simulink model "main"  (R2017b)
settings: Solver=FixedStepAuto  StartTime=0.0  StopTime=250  FixedStep=Ts  RelTol=1e-3
values from neighbouring files (symbols this model uses):
  dz = -0.1690    (= -0.169)    [prepareWorkspace.m]
  K = antisway.lqr()    [prepareWorkspace.m]
  omega_l = 4*2*pi    (= 25.1327412287)    [prepareWorkspace.m]
  omega_q = 1*2*pi    (= 6.28318530718)    [prepareWorkspace.m]
  Ts = 0.005    [prepareWorkspace.m]
  zeta_l = 0.7    [prepareWorkspace.m]
  zeta_q = 0.7    [prepareWorkspace.m]
undefined symbols (not defined in the file or in its folder): DiscIntNeverNeededParam, lambda, P0, Q, R, sigma, w0, x0
libraries: hydro x2
settings Model: Creator=motionlab  LastModifiedBy=motionlab
settings OptimizationCC: LocalBlockOutputs=off
settings DebuggingCC: BusObjectLabelMismatch=error
settings RTWCC: SystemTargetFile=TwinCAT.tlc  GenCodeOnly=on  MakeCommand=make_tct  TemplateMakefile=tct_msbuild.tmf  Description=TwinCAT Target  GenerateReport=on  TargetLang=C++
settings STFCustomTargetCC: TargetLangStandard=C++03 (ISO)  CompOptLevelCompliant=on  MATLABClassNameForMDSCustomization=Simulink.SoftwareTarget.TargetSpecificTriggerConfigurationBase  SystemTargetFile=TwinCAT.tlc
settings ConfigComp: PLC_TargetIDE=twincat3  PLC_GenerateReusableCode=on  PLC_InlineNamedConstant=on  PLC_ReuseMLFcnVariable=on  PLC_GenerateReport=off  PLC_LaunchReport=off

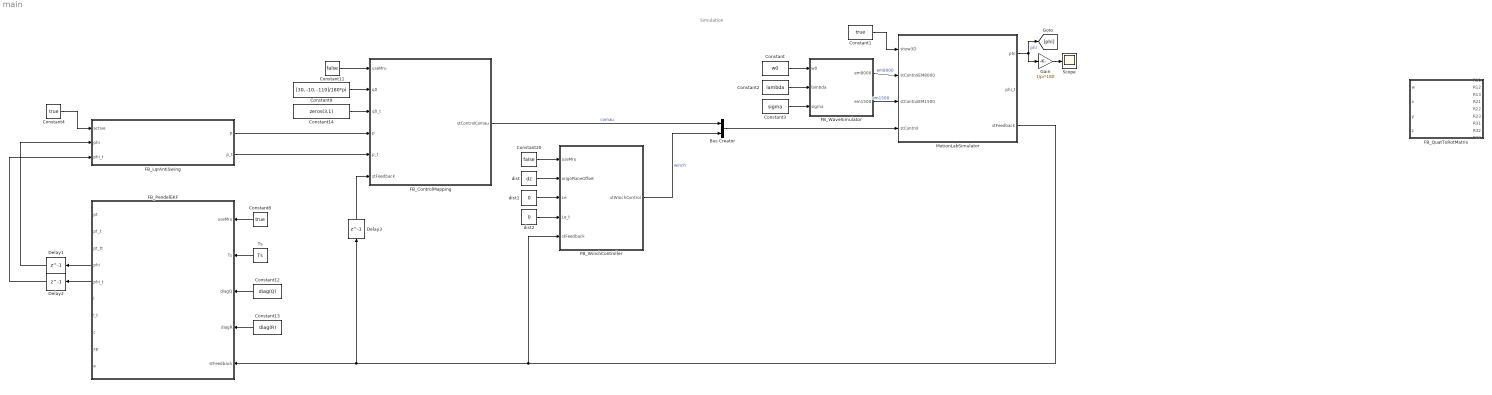
== system main ==
  note: Simulation
  Bus Creator : BusCreator  Inputs=2  OutDataTypeStr=Bus: ST_Control
  Constant : Constant  Value=w0
  Constant1 : Constant  Value=true
  Constant11 : Constant  Value=false
  Constant12 : Constant  Value=diag(Q)
  Constant13 : Constant  Value=diag(R)
  Constant14 : Constant  Value=zeros(3,1)
  Constant2 : Constant  Value=lambda
  Constant20 : Constant  Value=false
  Constant3 : Constant  Value=sigma
  Constant4 : Constant  Value=true
  Constant8 : Constant  Value=true
  Constant9 : Constant  Value=[30, -10, -110]/180*pi
  Delay1 : Delay  DelayLength=1
  Delay2 : Delay  DelayLength=1
  Delay3 : Delay  DelayLength=1
  FB_ControlMapping : MATLAB Function  TreatAsAtomicUnit=on
  FB_LqrAntiSwing : Subsystem  mask{lqrK=K, lqrMax=0.4}
      mask prompts: lqrK "LQR Gain"; lqrMax "LQR Saturation"
  FB_PendelEKF : Subsystem  TreatAsAtomicUnit=on  mask{ekfX0=x0}
      mask prompts: ekfX0 "x0"
      mask DialogControl Container3 Prompt: EKF Parmeters
  FB_QuatToRotMatrix : MATLAB Function  TreatAsAtomicUnit=on
  FB_WaveSimulator : Subsystem  TreatAsAtomicUnit=on
  FB_WinchController : Subsystem  TreatAsAtomicUnit=on
  Gain : Gain  Gain=1/pi*180
  MotionLabSimulator : Subsystem  mask{w_joints=omega_q, zeta_joints=zeta_q, w_winch=omega_l, zeta_winch=zeta_l, dz=dz, c=0.5, enableMruNoise=false}
      mask prompts: w_joints "omega [rad]"; zeta_joints "zeta [-]"; w_winch "omega [rad]"; zeta_winch "zeta [-]"; enableMruNoise "Enable"
      mask DialogControl ParameterGroupVar Prompt: Robot Joint Dynamics
      mask DialogControl Container3 Prompt: Winch Dynamics
      mask DialogControl Container4 Prompt: Ship Deck Offset From {b2}
      mask DialogControl Container5 Prompt: Pendulum Paramaters
      mask DialogControl Container6 Prompt: MRU Noise Simulation
  Scope : Scope
  Ts : Constant  Value=Ts
  dist : Constant  Value=dz
  dist1 : Constant  Value=0
  dist2 : Constant  Value=0
  wires:
  Constant1/1 -> MotionLabSimulator/1(show3D)
  Constant/1 -> FB_WaveSimulator/1(w0)
  Constant2/1 -> FB_WaveSimulator/2(lambda)
  Constant3/1 -> FB_WaveSimulator/3(sigma)
  MotionLabSimulator/1(phi) -> Gain/1, [phi]  "phi"
  Gain/1 -> Scope/1
  Constant20/1 -> FB_WinchController/1(useMru)
  dist/1 -> FB_WinchController/2(origoPlaneOffset)
  dist1/1 -> FB_WinchController/3(Le)
  FB_WaveSimulator/1(em8000) -> MotionLabSimulator/2(stControlEM8000)  "em8000"
  FB_WaveSimulator/2(em1500) -> MotionLabSimulator/3(stControlEM1500)  "em1500"
  Bus Creator/1 -> MotionLabSimulator/4(stControl)
  Constant9/1 -> FB_ControlMapping/2(q0)
  Constant11/1 -> FB_ControlMapping/1(useMru)
  Constant14/1 -> FB_ControlMapping/3(q0_t)
  FB_ControlMapping/1(stControlComau) -> Bus Creator/1  "comau"
  FB_WinchController/1(stWinchControl) -> Bus Creator/2  "winch"
  dist2/1 -> FB_WinchController/4(Le_t)
  MotionLabSimulator/3(stFeedback) -> FB_WinchController/5(stFeedback), Delay3/1, FB_PendelEKF/5(stFeedback)
  Delay3/1 -> FB_ControlMapping/6(stFeedback)
  FB_PendelEKF/5(phi_t) -> Delay2/1
  Constant8/1 -> FB_PendelEKF/1(useMru)
  Ts/1 -> FB_PendelEKF/2(Ts)
  FB_PendelEKF/4(phi) -> Delay1/1
  Constant12/1 -> FB_PendelEKF/3(diagQ)
  Constant13/1 -> FB_PendelEKF/4(diagR)
  Delay1/1 -> FB_LqrAntiSwing/2(phi)
  Delay2/1 -> FB_LqrAntiSwing/3(phi_t)
  Constant4/1 -> FB_LqrAntiSwing/1(active)
  FB_LqrAntiSwing/1(p) -> FB_ControlMapping/4(p)
  FB_LqrAntiSwing/2(p_t) -> FB_ControlMapping/5(p_t)

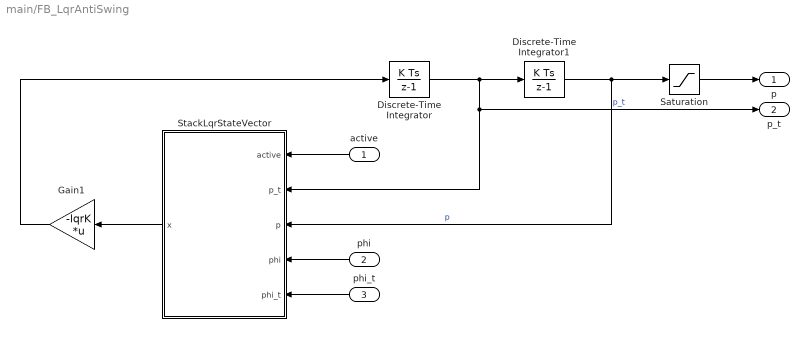
== system main/FB_LqrAntiSwing ==
  active : Inport
  phi : Inport  Port=2
  phi_t : Inport  Port=3
  Discrete-Time Integrator : DiscreteIntegrator  InitialCondition=zeros(3,1)  InitialConditionSetting=State (most efficient)  SampleTime=-1  ICPrevOutput=DiscIntNeverNeededParam  ICPrevScaledInput=DiscIntNeverNeededParam
  Discrete-Time Integrator1 : DiscreteIntegrator  InitialCondition=zeros(3,1)  InitialConditionSetting=State (most efficient)  SampleTime=-1  ICPrevOutput=DiscIntNeverNeededParam  ICPrevScaledInput=DiscIntNeverNeededParam
  Gain1 : Gain  Gain=-lqrK  Multiplication=Matrix(K*u)
  Saturation : Saturate  UpperLimit=abs(lqrMax)  LowerLimit=-abs(lqrMax)
  StackLqrStateVector : MATLAB Function  TreatAsAtomicUnit=on
  p : Outport
  p_t : Outport  Port=2
  wires:
  StackLqrStateVector/1(x) -> Gain1/1
  Gain1/1 -> Discrete-Time Integrator/1
  active/1 -> StackLqrStateVector/1(active)
  Discrete-Time Integrator1/1 -> StackLqrStateVector/3(p), Saturation/1  "p"
  Saturation/1 -> p/1
  Discrete-Time Integrator/1 -> Discrete-Time Integrator1/1, p_t/1, StackLqrStateVector/2(p_t)  "p_t"
  phi/1 -> StackLqrStateVector/4(phi)
  phi_t/1 -> StackLqrStateVector/5(phi_t)

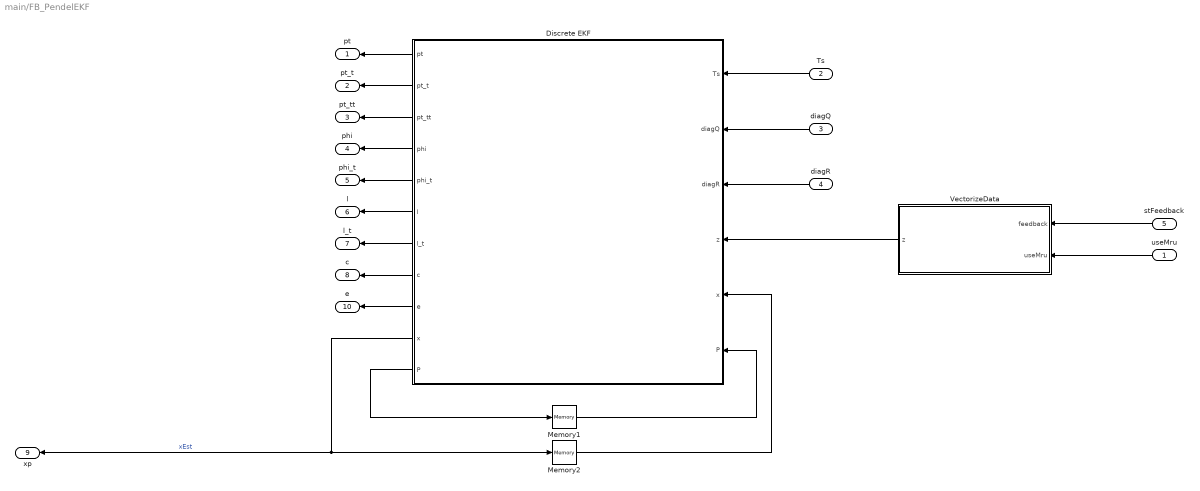
== system main/FB_PendelEKF ==
  useMru : Inport
  Ts : Inport  Port=2
  diagQ : Inport  Port=3
  diagR : Inport  Port=4
  stFeedback : Inport  Port=5  OutDataTypeStr=Bus: ST_Feedback
  Discrete EKF : MATLAB Function  TreatAsAtomicUnit=on
  Memory1 : Memory  InitialCondition=P0
  Memory2 : Memory  InitialCondition=ekfX0
  VectorizeData : MATLAB Function  TreatAsAtomicUnit=on
  pt : Outport
  pt_t : Outport  Port=2
  pt_tt : Outport  Port=3
  phi : Outport  Port=4
  phi_t : Outport  Port=5
  l : Outport  Port=6
  l_t : Outport  Port=7
  c : Outport  Port=8
  xp : Outport  Port=9
  e : Outport  Port=10
  wires:
  VectorizeData/1(z) -> Discrete EKF/4(z)
  Memory2/1 -> Discrete EKF/5("x ")
  Discrete EKF/11(P) -> Memory1/1
  Memory1/1 -> Discrete EKF/6("P ")
  diagR/1 -> Discrete EKF/3(diagR)
  diagQ/1 -> Discrete EKF/2(diagQ)
  Ts/1 -> Discrete EKF/1(Ts)
  Discrete EKF/10(x) -> xp/1, Memory2/1  "xEst"
  stFeedback/1 -> VectorizeData/1(feedback)
  useMru/1 -> VectorizeData/2(useMru)
  Discrete EKF/4(phi) -> phi/1
  Discrete EKF/5(phi_t) -> phi_t/1
  Discrete EKF/1(pt) -> pt/1
  Discrete EKF/2(pt_t) -> pt_t/1
  Discrete EKF/3(pt_tt) -> pt_tt/1
  Discrete EKF/6(l) -> l/1
  Discrete EKF/7(l_t) -> l_t/1
  Discrete EKF/8(c) -> c/1
  Discrete EKF/9(e) -> e/1

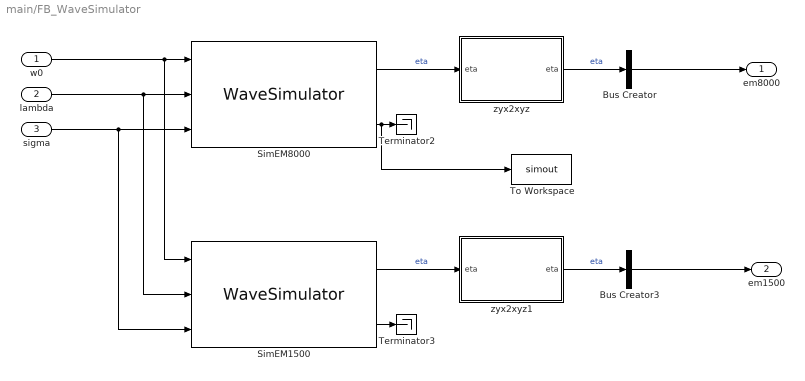
== system main/FB_WaveSimulator ==
  w0 : Inport
  lambda : Inport  Port=2
  sigma : Inport  Port=3
  Bus Creator : BusCreator  Inputs=1  OutDataTypeStr=Bus: ST_ControlStewart
  Bus Creator3 : BusCreator  Inputs=1  OutDataTypeStr=Bus: ST_ControlStewart
  SimEM1500 : hydro/WaveSimulator  poles=-30  seed=[5000,400,0,9000,150,42]  K1=1e4  K2=1e4  K3=1e8  K4=1e7  K5=1e8  K6=1e3  maxOutput=[0.1, 0.1, 0.3, 5/180*pi, 5/180*pi, 5/180*pi]  limitK=zeros(6,1)
      settings: SourceProductName=Hydro Library
  SimEM8000 : hydro/WaveSimulator  poles=-30  seed=[0,20,500,9000,400,200]  K1=1e4  K2=1e4  K3=1e8  K4=1e7  K5=1e8  K6=1e3  maxOutput=[0.1, 0.1, 0.4, 5/180*pi, 5/180*pi, 5/180*pi]  limitK=zeros(6,1)
      settings: SourceProductName=Hydro Library
  Terminator2 : Terminator
  Terminator3 : Terminator
  To Workspace : ToWorkspace  VariableName=simout  SaveFormat=Timeseries  SampleTime=-1
  zyx2xyz : MATLAB Function  TreatAsAtomicUnit=on
  zyx2xyz1 : MATLAB Function  TreatAsAtomicUnit=on
  em8000 : Outport
  em1500 : Outport  Port=2
  wires:
  zyx2xyz/1(eta) -> Bus Creator/1  "eta"
  Bus Creator3/1 -> em1500/1
  Bus Creator/1 -> em8000/1
  zyx2xyz1/1(eta) -> Bus Creator3/1  "eta"
  SimEM1500/1 -> zyx2xyz1/1("eta ")  "eta"
  SimEM8000/2 -> To Workspace/1, Terminator2/1
  SimEM8000/1 -> zyx2xyz/1("eta ")  "eta"
  SimEM1500/2 -> Terminator3/1
  w0/1 -> SimEM8000/1, SimEM1500/1
  lambda/1 -> SimEM8000/2, SimEM1500/2
  sigma/1 -> SimEM8000/3, SimEM1500/3

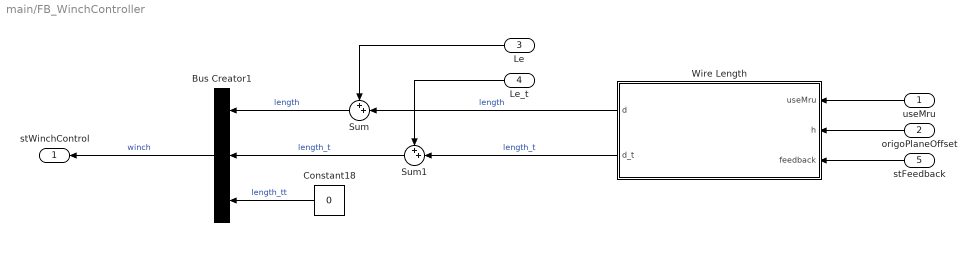
== system main/FB_WinchController ==
  useMru : Inport
  origoPlaneOffset : Inport  Port=2
  Le : Inport  Port=3
  Le_t : Inport  Port=4
  stFeedback : Inport  Port=5
  Bus Creator1 : BusCreator  Inputs=3  OutDataTypeStr=Bus: ST_ControlWinch
  Constant18 : Constant  Value=0
  Sum : Sum  Inputs=++|
  Sum1 : Sum  Inputs=++|
  Wire Length : MATLAB Function  TreatAsAtomicUnit=on
  stWinchControl : Outport
  wires:
  Bus Creator1/1 -> stWinchControl/1  "winch"
  useMru/1 -> Wire Length/1(useMru)
  origoPlaneOffset/1 -> Wire Length/2(h)
  Constant18/1 -> Bus Creator1/3  "length_tt"
  Sum/1 -> Bus Creator1/1  "length"
  Wire Length/1(d) -> Sum/2  "length"
  Le/1 -> Sum/1
  stFeedback/1 -> Wire Length/3(feedback)
  Sum1/1 -> Bus Creator1/2  "length_t"
  Wire Length/2(d_t) -> Sum1/2  "length_t"
  Le_t/1 -> Sum1/1

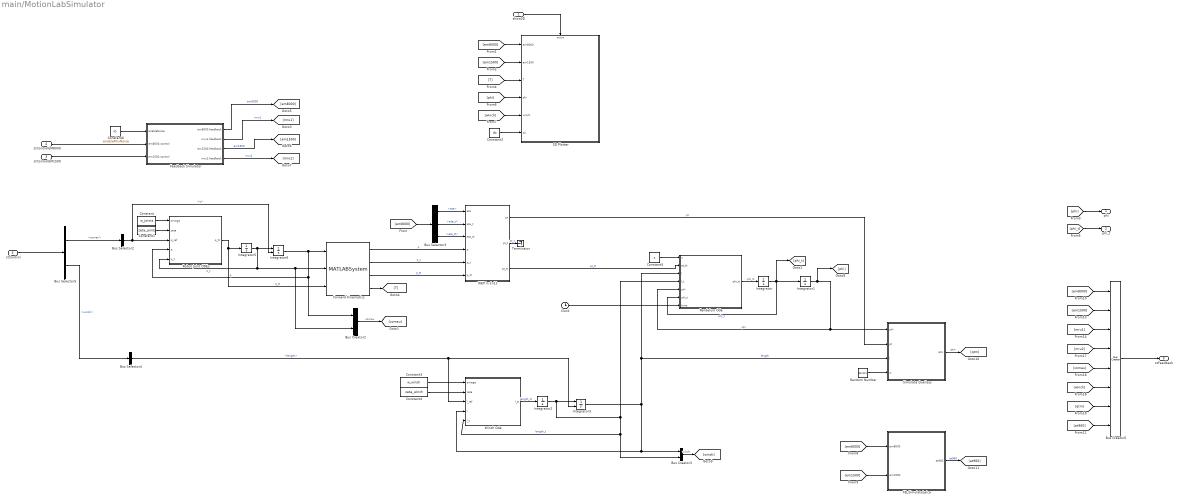
== system main/MotionLabSimulator ==
  show3D : Inport
  stControlEM8000 : Inport  Port=2  OutDataTypeStr=Bus: ST_ControlStewart
  stControlEM1500 : Inport  Port=3  OutDataTypeStr=Bus: ST_ControlStewart
  stControl : Inport  Port=4  OutDataTypeStr=Bus: ST_Control
  3D Plotter : Subsystem
  Bus Creator2 : BusCreator  Inputs=2  OutDataTypeStr=Bus: ST_FeedbackComau
  Bus Creator3 : BusCreator  Inputs=2  OutDataTypeStr=Bus: ST_FeedbackWinch
  Bus Creator5 : BusCreator  Inputs=8  OutDataTypeStr=Bus: ST_Feedback
  Bus Selector2 : BusSelector  OutputSignals=q
  Bus Selector3 : BusSelector  OutputSignals=eta,eta_t,eta_tt
  Bus Selector4 : BusSelector  OutputSignals=length
  Bus Selector5 : BusSelector  OutputSignals=comau,winch
  Clock : Clock
  Constant : Constant  Value=w_joints
  Constant1 : Constant  Value=zeta_joints
  Constant2 : Constant  Value=dz
  Constant3 : Constant  Value=w_winch
  Constant4 : Constant  Value=zeta_winch
  Constant5 : Constant  Value=c
  Constant6 : Constant  Value=enableMruNoise
  FB_SimulateLeica : MATLAB Function  TreatAsAtomicUnit=on
  Feedback Simulator : Subsystem
  Forward Kinematics : MATLABSystem  System=motionlab.ComauRobot3DOF  fk=on  outputT=on  SimulateUsing=Interpreted execution
      mask Type: motionlab.ComauRobot3DOF
      mask Display:
      | disp('ComauRobot3DOF');
      | port_label('input',1,'q');
      | port_label('input',2,'q_t');
      | port_label('input',3,'q_tt');
      | port_label('output',1,'p');
      | port_label('output',2,'p_t');
      | port_label('output',3,'p_tt');
      | port_label('output',4,'T');
  Integrator : Integrator  InitialCondition=zeros(2,1)
  Integrator1 : Integrator  InitialCondition=zeros(2,1)
  Integrator2 : Integrator
  Integrator3 : Integrator  InitialConditionSource=external
  Integrator5 : Integrator  InitialCondition=zeros(3,1)
  Integrator6 : Integrator  InitialConditionSource=external  InitialCondition=zeros(3,1)
  Pendelum Ode : MATLAB Function  TreatAsAtomicUnit=on  SystemSampleTime=Ts
  Random Number : RandomNumber  Variance=[1, 1, 1, 1]*0  Seed=[0, 500, 1000, 1200]  SampleTime=Ts
  Robot Joint ODEs : MATLAB Function  TreatAsAtomicUnit=on
  Simulate Qualisys : MATLAB Function  TreatAsAtomicUnit=on
  Terminator : Terminator
  "WEP in {n1}" : MATLAB Function  TreatAsAtomicUnit=on
  Winch Ode : MATLAB Function  TreatAsAtomicUnit=on
  phi : Outport
  phi_t : Outport  Port=2
  stFeedback : Outport  Port=3  OutDataTypeStr=Bus: ST_Feedback
  wires:
  [mru1] -> Bus Creator5/3
  [winch] -> 3D Plotter/5(winch)
  [mru2] -> Bus Creator5/4
  [em1500] -> Bus Creator5/2
  [em8000] -> Bus Creator5/1
  Bus Creator3/1 -> [winch]  "winch"
  Bus Creator5/1 -> stFeedback/1
  [qtm] -> Bus Creator5/7
  [comau] -> Bus Creator5/5
  [winch] -> Bus Creator5/6
  "WEP in {n1}"/2(pt_t) -> Terminator/1  "pt_t"
  Winch Ode/1(l_tt) -> Integrator2/1  "length_tt"
  show3D/1 -> 3D Plotter/Enable
  Integrator/1 -> [phi_t], Integrator1/1, Pendelum Ode/6(phi_t)  "phi_t"
  "WEP in {n1}"/3(pt_tt) -> Pendelum Ode/2(pt_tt)  "pt_tt"
  Forward Kinematics/4 -> [T]
  Bus Selector2/1 -> Integrator6/2, Robot Joint ODEs/3(q_ref)  "<q>"
  Pendelum Ode/1(phi_tt) -> Integrator/1  "phi_tt"
  Integrator3/1 -> Bus Creator3/1, Winch Ode/4(l), Simulate Qualisys/3(l), Pendelum Ode/3(l)  "length"
  Integrator2/1 -> Pendelum Ode/4(l_t), Winch Ode/5(l_t), Bus Creator3/2, Integrator3/1  "length_t"
  Integrator1/1 -> [phi], Pendelum Ode/5(phi), Simulate Qualisys/1(phi)  "phi"
  Robot Joint ODEs/1(q_tt) -> Integrator5/1, Forward Kinematics/3  "q_tt"
  Integrator5/1 -> Robot Joint ODEs/5(q_t), Forward Kinematics/2, Bus Creator2/2, Integrator6/1  "q_t"
  Integrator6/1 -> Bus Creator2/1, Robot Joint ODEs/4(q), Forward Kinematics/1  "q"
  Forward Kinematics/1 -> "WEP in {n1}"/4(p)  "p"
  Forward Kinematics/2 -> "WEP in {n1}"/5(p_t)  "p_t"
  Forward Kinematics/3 -> "WEP in {n1}"/6(p_tt)  "p_tt"
  Simulate Qualisys/1(qtm) -> [qtm]  "qtm"
  Bus Selector4/1 -> Integrator3/2, Winch Ode/3(l_ref)  "<length>"
  stControl/1 -> Bus Selector5/1
  Bus Selector3/1 -> "WEP in {n1}"/1(eta)  "<eta>"
  Bus Selector3/3 -> "WEP in {n1}"/3(eta_tt)  "<eta_tt>"
  Bus Selector3/2 -> "WEP in {n1}"/2(eta_t)  "<eta_t>"
  "WEP in {n1}"/1(pt) -> Simulate Qualisys/2(pt)  "pt"
  Feedback Simulator/1(em8000.feedback) -> [em8000]  "em8000"
  [phi] -> 3D Plotter/4(phi)
  Feedback Simulator/3(em1500.feedback) -> [em1500]  "em1500"
  [em8000] -> Bus Selector3/1
  [em1500] -> 3D Plotter/2(em1500)
  Feedback Simulator/2(mru1.feedback) -> [mru1]  "mru1"
  [em8000] -> 3D Plotter/1(em8000)
  Bus Creator2/1 -> [comau]  "comau"
  Feedback Simulator/4(mru2.feedback) -> [mru2]  "mru2"
  [T] -> 3D Plotter/3(T)
  [phi] -> phi/1
  Constant/1 -> Robot Joint ODEs/1(omega)
  Constant1/1 -> Robot Joint ODEs/2(zeta)
  Constant2/1 -> 3D Plotter/6(dz)
  Constant3/1 -> Winch Ode/1(omega)
  Constant4/1 -> Winch Ode/2(zeta)
  Constant5/1 -> Pendelum Ode/1(c)
  [phi_t] -> phi_t/1
  Constant6/1 -> Feedback Simulator/1(enableNoise)
  Random Number/1 -> Simulate Qualisys/4(w)
  [em8000] -> FB_SimulateLeica/1(em8000)
  [em1500] -> FB_SimulateLeica/2(em1500)
  FB_SimulateLeica/1(at960) -> [at960]  "at960"
  [at960] -> Bus Creator5/8
  Bus Selector5/1 -> Bus Selector2/1  "<comau>"
  Bus Selector5/2 -> Bus Selector4/1  "<winch>"
  Clock/1 -> Pendelum Ode/7(time)
  stControlEM8000/1 -> Feedback Simulator/2(em8000.control)
  stControlEM1500/1 -> Feedback Simulator/3(em1500.control)

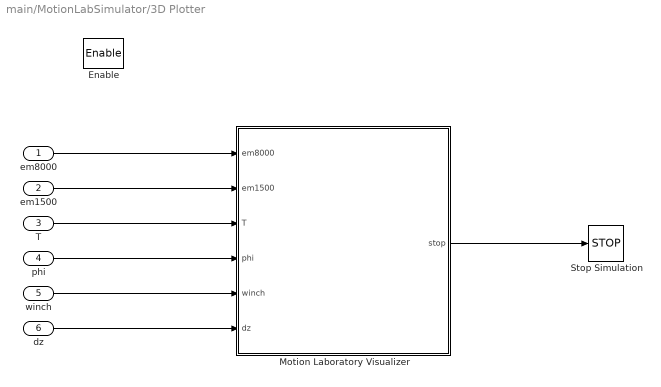
== system main/MotionLabSimulator/3D Plotter ==
  em8000 : Inport
  em1500 : Inport  Port=2
  T : Inport  Port=3
  phi : Inport  Port=4
  winch : Inport  Port=5
  dz : Inport  Port=6
  Enable : EnablePort
  Motion Laboratory Visualizer : MATLAB Function  TreatAsAtomicUnit=on  SystemSampleTime=0.1
  Stop Simulation : Stop
  wires:
  em8000/1 -> Motion Laboratory Visualizer/1(em8000)
  phi/1 -> Motion Laboratory Visualizer/4(phi)
  winch/1 -> Motion Laboratory Visualizer/5(winch)
  em1500/1 -> Motion Laboratory Visualizer/2(em1500)
  T/1 -> Motion Laboratory Visualizer/3(T)
  Motion Laboratory Visualizer/1(stop) -> Stop Simulation/1
  dz/1 -> Motion Laboratory Visualizer/6(dz)

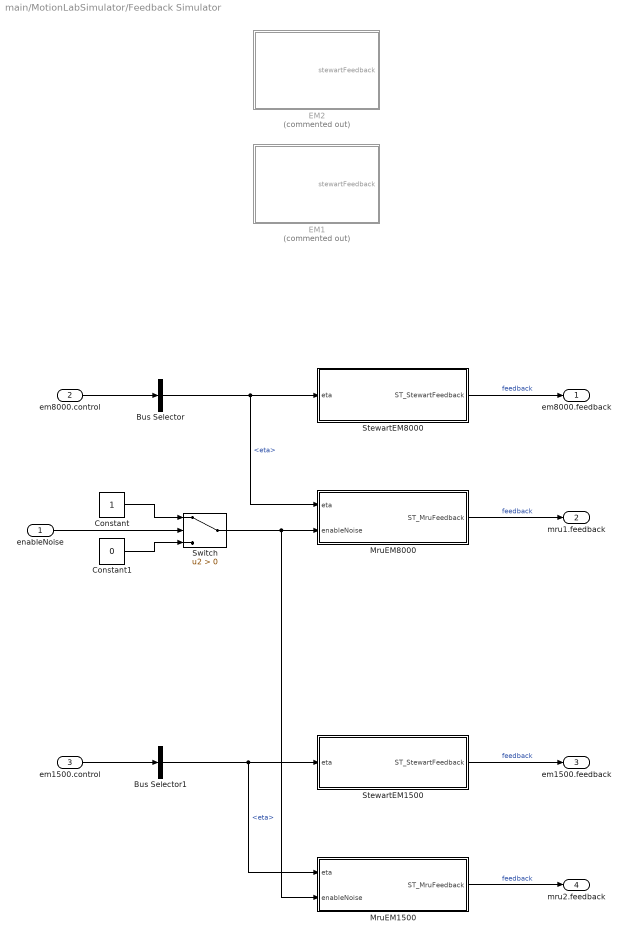
== system main/MotionLabSimulator/Feedback Simulator ==
  enableNoise : Inport
  em8000.control : Inport  Port=2  OutDataTypeStr=Bus: ST_ControlStewart
  em1500.control : Inport  Port=3  OutDataTypeStr=Bus: ST_ControlStewart
  Bus Selector : BusSelector  OutputSignals=eta
  Bus Selector1 : BusSelector  OutputSignals=eta
  Constant : Constant
  Constant1 : Constant  Value=0
  EM1 : Subsystem  Commented=on  TreatAsAtomicUnit=on  mask{A_surge=0.2, f_surge=0.1, phase_surge=0, A_sway=0.2, f_sway=0.05, phase_sway=200, A_heave=0.4, f_heave=0.12, phase_heave=30, A_phi=5.0, f_phi=0.09, phase_phi=45, A_theta=5.0, f_theta=0.15, phase_theta=60, A_psi=5.0, f_psi=0.12, phase_psi=-40}
      mask prompts: A_surge "Amplitude [m]"; f_surge "Frequency [Hz]"; phase_surge "Phase [deg]"; A_sway "Amplitude [m]"; f_sway "Frequency [Hz]"; phase_sway "Phase [deg]"; A_heave "Amplitude [m]"; f_heave "Frequency [Hz]"; phase_heave "Phase [deg]"; A_phi "Amplitude [deg]"; f_phi "Frequency [Hz]"; phase_phi "Phase [deg]"; A_theta "Amplitude [deg]"; f_theta "Frequency [Hz]"; phase_theta "Phase [deg]"; A_psi "Amplitude [deg]"; f_psi "Frequency [Hz]"; phase_psi "Phase [deg]"
      mask DialogControl ParameterGroupVar Prompt: Surge
      mask DialogControl Container3 Prompt: Sway
      mask DialogControl Container4 Prompt: Heave
      mask DialogControl Container5 Prompt: Phi
      mask DialogControl Container6 Prompt: Theta
      mask DialogControl Container7 Prompt: Psi
  EM2 : Subsystem  Commented=on  TreatAsAtomicUnit=on  mask{A_surge=0.05, f_surge=0.1, phase_surge=0, A_sway=0.05, f_sway=0.12, phase_sway=120, A_heave=0.4, f_heave=0.12, phase_heave=30, A_phi=5, f_phi=0.09, phase_phi=45, A_theta=5, f_theta=0.15, phase_theta=60, A_psi=5, f_psi=0.12, phase_psi=-40}
      mask prompts: A_surge "Amplitude [m]"; f_surge "Frequency [Hz]"; phase_surge "Phase [deg]"; A_sway "Amplitude [m]"; f_sway "Frequency [Hz]"; phase_sway "Phase [deg]"; A_heave "Amplitude [m]"; f_heave "Frequency [Hz]"; phase_heave "Phase [deg]"; A_phi "Amplitude [deg]"; f_phi "Frequency [Hz]"; phase_phi "Phase [deg]"; A_theta "Amplitude [deg]"; f_theta "Frequency [Hz]"; phase_theta "Phase [deg]"; A_psi "Amplitude [deg]"; f_psi "Frequency [Hz]"; phase_psi "Phase [deg]"
      mask DialogControl ParameterGroupVar Prompt: Surge
      mask DialogControl Container3 Prompt: Sway
      mask DialogControl Container4 Prompt: Heave
      mask DialogControl Container5 Prompt: Phi
      mask DialogControl Container6 Prompt: Theta
      mask DialogControl Container7 Prompt: Psi
  MruEM1500 : Subsystem
  MruEM8000 : Subsystem
  StewartEM1500 : Subsystem
  StewartEM8000 : Subsystem
  Switch : Switch  Criteria=u2 > Threshold
  em8000.feedback : Outport
  mru1.feedback : Outport  Port=2
  em1500.feedback : Outport  Port=3
  mru2.feedback : Outport  Port=4
  wires:
  Switch/1 -> MruEM1500/2(enableNoise), MruEM8000/2(enableNoise)
  StewartEM8000/1(ST_StewartFeedback) -> em8000.feedback/1  "feedback"
  MruEM8000/1(ST_MruFeedback) -> mru1.feedback/1  "feedback"
  StewartEM1500/1(ST_StewartFeedback) -> em1500.feedback/1  "feedback"
  MruEM1500/1(ST_MruFeedback) -> mru2.feedback/1  "feedback"
  em8000.control/1 -> Bus Selector/1
  Bus Selector/1 -> MruEM8000/1(eta), StewartEM8000/1(eta)  "<eta>"
  em1500.control/1 -> Bus Selector1/1
  Bus Selector1/1 -> MruEM1500/1(eta), StewartEM1500/1(eta)  "<eta>"
  enableNoise/1 -> Switch/2
  Constant/1 -> Switch/1
  Constant1/1 -> Switch/3

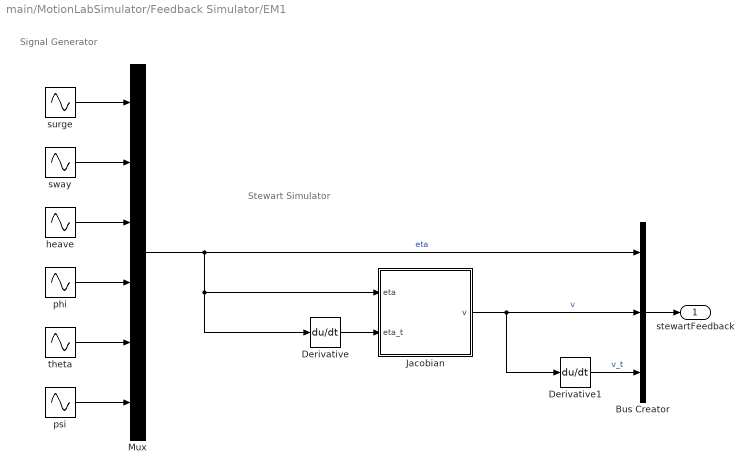
== system main/MotionLabSimulator/Feedback Simulator/EM1 ==
  note: Signal Generator
  note: Stewart Simulator
  Bus Creator : BusCreator  Inputs=3  OutDataTypeStr=Bus: StewartFeedback
  Derivative : Derivative
  Derivative1 : Derivative
  Jacobian : MATLAB Function  TreatAsAtomicUnit=on
  Mux : Mux  Inputs=6
  heave : Sin  Amplitude=A_heave  Frequency=f_heave*2*pi  Phase=phase_heave/180*pi
  phi : Sin  Amplitude=A_phi/180*pi  Frequency=f_phi*2*pi  Phase=phase_phi/180*pi
  psi : Sin  Amplitude=A_psi/180*pi  Frequency=f_psi*2*pi  Phase=phase_psi/180*pi
  surge : Sin  Amplitude=A_surge  Frequency=f_surge*2*pi  Phase=phase_surge/180*pi
  sway : Sin  Amplitude=A_sway  Frequency=f_sway*2*pi  Phase=phase_sway/180*pi
  theta : Sin  Amplitude=A_theta/180*pi  Frequency=f_theta*2*pi  Phase=phase_theta/180*pi
  stewartFeedback : Outport  OutDataTypeStr=Bus: StewartFeedback
  wires:
  psi/1 -> Mux/6
  phi/1 -> Mux/4
  sway/1 -> Mux/2
  theta/1 -> Mux/5
  surge/1 -> Mux/1
  heave/1 -> Mux/3
  Jacobian/1(v) -> Derivative1/1, Bus Creator/2  "v"
  Mux/1 -> Bus Creator/1, Derivative/1, Jacobian/1(eta)  "eta"
  Derivative/1 -> Jacobian/2(eta_t)
  Derivative1/1 -> Bus Creator/3  "v_t"
  Bus Creator/1 -> stewartFeedback/1

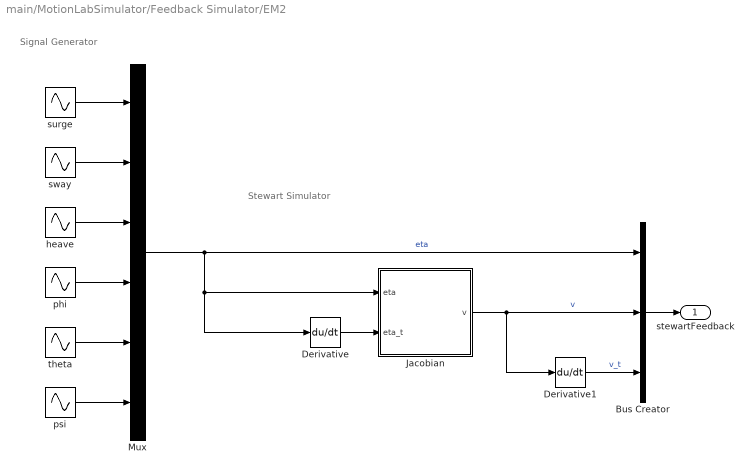
== system main/MotionLabSimulator/Feedback Simulator/EM2 ==
  note: Signal Generator
  note: Stewart Simulator
  Bus Creator : BusCreator  Inputs=3  OutDataTypeStr=Bus: StewartFeedback
  Derivative : Derivative
  Derivative1 : Derivative  CoefficientInTFapproximation=-1
  Jacobian : MATLAB Function  TreatAsAtomicUnit=on
  Mux : Mux  Inputs=6
  heave : Sin  Amplitude=A_heave  Frequency=f_heave*2*pi  Phase=phase_heave/180*pi
  phi : Sin  Amplitude=A_phi/180*pi  Frequency=f_phi*2*pi  Phase=phase_phi/180*pi
  psi : Sin  Amplitude=A_psi/180*pi  Frequency=f_psi*2*pi  Phase=phase_psi/180*pi
  surge : Sin  Amplitude=A_surge  Frequency=f_surge*2*pi  Phase=phase_surge/180*pi
  sway : Sin  Amplitude=A_sway  Frequency=f_sway*2*pi  Phase=phase_sway/180*pi
  theta : Sin  Amplitude=A_theta/180*pi  Frequency=f_theta*2*pi  Phase=phase_theta/180*pi
  stewartFeedback : Outport  OutDataTypeStr=Bus: StewartFeedback
  wires:
  psi/1 -> Mux/6
  phi/1 -> Mux/4
  sway/1 -> Mux/2
  theta/1 -> Mux/5
  surge/1 -> Mux/1
  heave/1 -> Mux/3
  Jacobian/1(v) -> Derivative1/1, Bus Creator/2  "v"
  Mux/1 -> Bus Creator/1, Derivative/1, Jacobian/1(eta)  "eta"
  Derivative/1 -> Jacobian/2(eta_t)
  Derivative1/1 -> Bus Creator/3  "v_t"
  Bus Creator/1 -> stewartFeedback/1

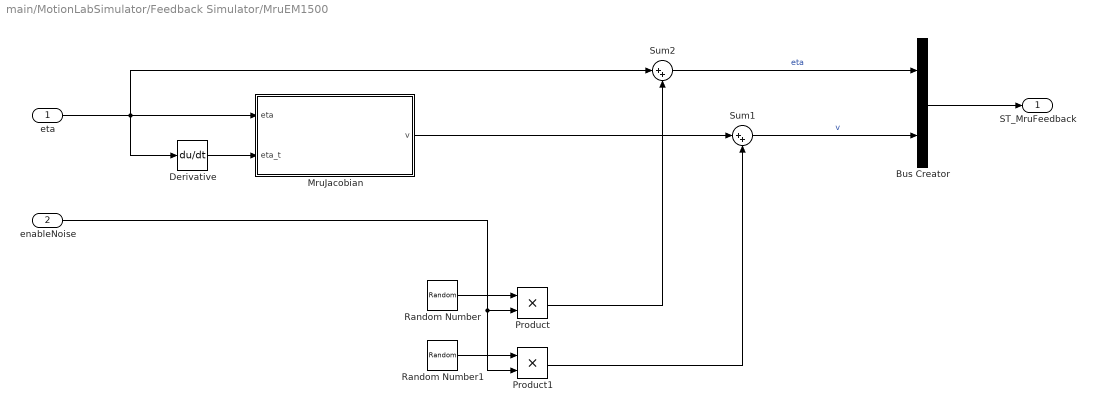
== system main/MotionLabSimulator/Feedback Simulator/MruEM1500 ==
  eta : Inport
  enableNoise : Inport  Port=2
  Bus Creator : BusCreator  Inputs=2  OutDataTypeStr=Bus: ST_FeedbackMru
  Derivative : Derivative
  MruJacobian : MATLAB Function  TreatAsAtomicUnit=on
  Product : Product
  Product1 : Product
  Random Number : RandomNumber  Variance=sim.mru1.var.eta  Seed=randi(100000, 6, 1)  SampleTime=Ts
  Random Number1 : RandomNumber  Variance=sim.mru1.var.v  Seed=randi(100000, 6, 1)  SampleTime=Ts
  Sum1 : Sum  Inputs=|++
  Sum2 : Sum  Inputs=|++
  ST_MruFeedback : Outport
  wires:
  Derivative/1 -> MruJacobian/2(eta_t)
  eta/1 -> Sum2/1, Derivative/1, MruJacobian/1(eta)
  MruJacobian/1(v) -> Sum1/1
  Sum1/1 -> Bus Creator/2  "v"
  Sum2/1 -> Bus Creator/1  "eta"
  Random Number/1 -> Product/1
  Product/1 -> Sum2/2
  Random Number1/1 -> Product1/1
  Product1/1 -> Sum1/2
  enableNoise/1 -> Product1/2, Product/2
  Bus Creator/1 -> ST_MruFeedback/1

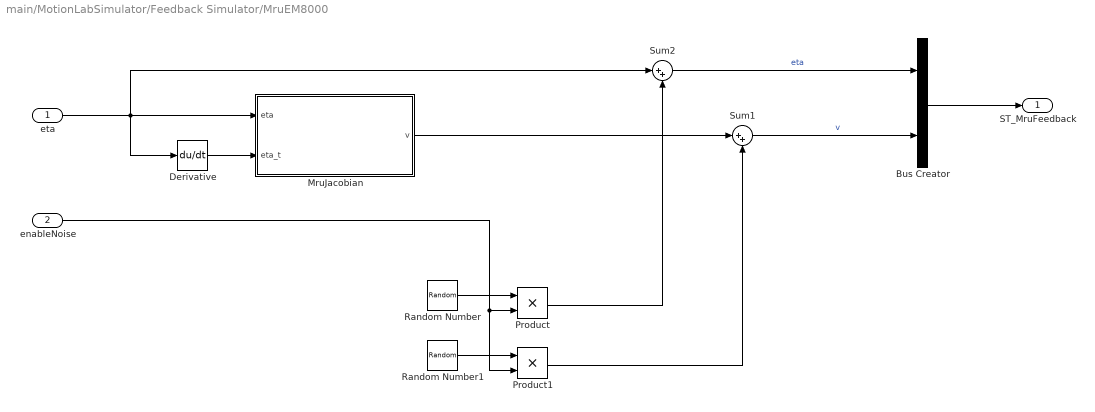
== system main/MotionLabSimulator/Feedback Simulator/MruEM8000 ==
  eta : Inport
  enableNoise : Inport  Port=2
  Bus Creator : BusCreator  Inputs=2  OutDataTypeStr=Bus: ST_FeedbackMru
  Derivative : Derivative
  MruJacobian : MATLAB Function  TreatAsAtomicUnit=on
  Product : Product
  Product1 : Product
  Random Number : RandomNumber  Variance=sim.mru1.var.eta  Seed=randi(100000, 6, 1)  SampleTime=Ts
  Random Number1 : RandomNumber  Variance=sim.mru1.var.v  Seed=randi(100000, 6, 1)  SampleTime=Ts
  Sum1 : Sum  Inputs=|++
  Sum2 : Sum  Inputs=|++
  ST_MruFeedback : Outport
  wires:
  Derivative/1 -> MruJacobian/2(eta_t)
  eta/1 -> Sum2/1, Derivative/1, MruJacobian/1(eta)
  MruJacobian/1(v) -> Sum1/1
  Sum1/1 -> Bus Creator/2  "v"
  Sum2/1 -> Bus Creator/1  "eta"
  Random Number/1 -> Product/1
  Product/1 -> Sum2/2
  Random Number1/1 -> Product1/1
  Product1/1 -> Sum1/2
  Bus Creator/1 -> ST_MruFeedback/1
  enableNoise/1 -> Product1/2, Product/2

== system main/MotionLabSimulator/Feedback Simulator/StewartEM1500 ==
  eta : Inport
  Bus Creator : BusCreator  Inputs=3  OutDataTypeStr=Bus: ST_FeedbackStewart
  Derivative2 : Derivative
  Derivative3 : Derivative  CoefficientInTFapproximation=-1
  ST_StewartFeedback : Outport
  wires:
  Derivative2/1 -> Bus Creator/2, Derivative3/1  "eta_t"
  Bus Creator/1 -> ST_StewartFeedback/1
  Derivative3/1 -> Bus Creator/3  "eta_tt"
  eta/1 -> Bus Creator/1, Derivative2/1  "eta"

== system main/MotionLabSimulator/Feedback Simulator/StewartEM8000 ==
  eta : Inport
  Bus Creator : BusCreator  Inputs=3  OutDataTypeStr=Bus: ST_FeedbackStewart
  Derivative2 : Derivative
  Derivative3 : Derivative  CoefficientInTFapproximation=-1
  ST_StewartFeedback : Outport
  wires:
  Derivative2/1 -> Bus Creator/2, Derivative3/1  "eta_t"
  Bus Creator/1 -> ST_StewartFeedback/1
  Derivative3/1 -> Bus Creator/3  "eta_tt"
  eta/1 -> Bus Creator/1, Derivative2/1  "eta"

== matlab function main/MotionLabSimulator/3D Plotter/Motion Laboratory Visualizer ==
  data: stop output; em8000 input; em1500 input; T input; phi input; winch input; dz input
function stop  = fcn(em8000, em1500, T, phi, winch, dz)

% Load calibration data
coderData = coder.load('+motionlab/calib.mat');
calib = coderData.calib;

% Load plot objects
%sphere = coder.load('spherePatch.mat');


% {g} -> {b1}
H1 = eye(4);
H1(1:3,4)= em8000.eta(1:3);
H1(1:3,1:3) = math3d.Rxyz(em8000.eta(4:6));

Hgn1 = calib.WORLD_TO_EM8000.H;
Hgb1 = Hgn1*H1;

% {g} -> {b2}
H2 = eye(4);
H2(1:3,4)= em1500.eta(1:3);
H2(1:3,1:3) = math3d.Rxyz(em1500.eta(4:6));

Hgn2 = calib.WORLD_TO_EM1500.H;
Hgb2 = Hgn2*H2;

% {b1} -> {r}
H1r = calib.EM8000_TO_COMAU.H;

% {r} -> {j1}
Hr1 = T(:,:,1);
Hr2 = Hr1*T(:,:,2);
Hr3 = Hr2*T(:,:,3);
Hrt = Hr3*T(:,:,4);



% Set up plot
persistent h;

% Declare plot3 as extrinsic
coder.extrinsic('plot3');


if isempty(h)
    close all
    
    h = figure('Name', 'Animation');
    hold on;
    grid on;
    axis equal;
    view([-40, 20]);
    
    
    % View limits
    xlim([-4, 2])
    ylim([-3, 3])
    zlim([0, 7])
    
    % Labels
    xlabel('x-axis')
    ylabel('y-axis')
    zlabel('z-axis')
    
    % Figure sizing
    screeenSz = [1920, 1200];
    figSz = [4, 3]/4*1200;
    set(h, 'Position', [
        screeenSz(1)/2 - figSz(1)/2
        screeenSz(2)/2 - figSz(2)/2
        figSz(1)
        figSz(2)
    ])
end

if ishandle(h)
    cla;
    
    % Ground coordinate system
    plotCoordinateSystem(eye(4));
    
    % EM8000
    plotCoordinateSystem(Hgn1);
    plotCoordinateSystem(Hgb1);
    
    % EM1500
    plotCoordinateSystem(Hgn2);
    plotCoordinateSystem(Hgb2);
    
    % Comau Robot Coordinates given in {g}
    Hgr = Hgb1*H1r;
    Hg1 = Hgr*Hr1;
    Hg2 = Hgr*Hr2;
    Hg3 = Hgr*Hr3;
    Hgt = Hgr*Hrt;
    
    Hgq = calib.WORLD_TO_QTM.H;
    
    % Hook position in {n1}   
    pt_n = Hgn1(1:3,1:3)'*Hgt(1:3,4);
    ph_n = pendel.kinematics(pt_n, phi, winch.length);
    
    ph = Hgn1(1:3,1:3)*ph_n;
    
    % Robot Coordinates
    plotCoordinateSystem(Hgr);
    plotCoordinateSystem(Hg1);
    plotCoordinateSystem(Hg2);
    plotCoordinateSystem(Hg3);
    plotCoordinateSystem(Hgt);
    
    % Qualisys coordinate
    plotCoordinateSystem(Hgq);
    
    % Links
    plotLine(Hgr(1:3,4), Hg1(1:3,4));
    plotLine(Hg1(1:3,4), Hg2(1:3,4));
    plotLine(Hg2(1:3,4), Hg3(1:3,4));
    plotLine(Hg3(1:3,4), Hgt(1:3,4));
    
    % Load
    plotLine(Hgt(1:3,4), ph);
    %plotLoadSphere(ph, sphere.fvc);
    
    % Plot ship plane
    plotPlane(Hgb2, dz);
    
%     % Projected point
%     Hn1t = math3d.InvH(Hgn1)*Hgt;
%     dir = [0; 0; 1];
%     pp = Hn1t(1:3,4) + d*dir;
%     p = Hgn1*[pp; 1];
%     plot3(p(1), p(2), p(3), 'k.')
    
      
    % Update plots
    drawnow;
end


% Close when figure is closed
stop = false;
if ~ishandle(h)
    stop = true;
end



end

function plotLine(p1, p2)
    link = zeros(2,3);
    link(1,:) = p1;
    link(2,:) = p2;
    
    plot3(link(:,1), link(:,2), link(:,3), 'k')
end

function plotLoadSphere(ph, fvc)
    coder.extrinsic('patch');

    % Patch data
    fvc.vertices(:,1) = fvc.vertices(:,1) + ph(1);
    fvc.vertices(:,2) = fvc.vertices(:,2) + ph(2);
    fvc.vertices(:,3) = fvc.vertices(:,3) + ph(3);
    
    patch('Faces', fvc.faces, 'Vertices', fvc.vertices, 'FaceColor', 'k')
    
end

function plotPlane(H, dz)

coder.extrinsic('patch');

x = 3/2;
y = 5/2;
z = dz;
xyPlane = [
    -x,  x,  x, -x
    -y, -y,  y,  y
     z,  z,  z,  z
     1,  1,  1,  1
];

plane = H*xyPlane;

patch(plane(1,:), plane(2,:), plane(3,:), 'r', 'FaceAlpha', 0.5);

end

function plotCoordinateSystem(varargin)
    % Rotation and translation
    H = varargin{1};
    t = H(1:3,4);
    R = H(1:3,1:3);

    % Axis colors
    colors = {'r', 'g', 'b'};

    % Plot all 3 axis
    axis = zeros(2,3);
    axLength = 0.4;
    for i = 1:3
        axis(1,:) = t;
        axis(2,:) = t + R(:,i)*axLength;

        plot3(axis(:,1), axis(:,2), axis(:,3), colors{i}, 'LineWidth', 1);
    end
    
    if nargin > 1
        loc = mean(axis);
        text(loc(1), loc(2), loc(3), varargin{2})
    end
end

== matlab function main/FB_WaveSimulator/zyx2xyz ==
  data: eta input; eta output
function eta = fcn(eta)

% Convert Angle sequence
eta(4:6) = math3d.zyx2xyz(eta(4:6));

end

== matlab function main/MotionLabSimulator/Feedback Simulator/MruEM1500/MruJacobian ==
  data: eta input; v output; eta_t input
function v = fcn(eta, eta_t)

% Velcoity Jacobian
J = eye(6);
J(4:6,4:6) = math3d.Tphi(eta(4:6), 'xyz');

% Body fixed velocities
v = J\eta_t;

end

== matlab function main/MotionLabSimulator/Pendelum Ode ==
  data: c input; phi_tt output; pt_tt input; l input; l_t input; phi input; phi_t input; time input
function phi_tt  = fcn(c, pt_tt, l, l_t, phi, phi_t, time)
% Paramaters
g = 9.81;


% if (time > 10) && (time < 10.5)
%     tau = [
%         1
%         0
%     ];
% elseif (time > 20) && (time < 20.5)
%     tau = [
%         0
%         1
%     ];
% else
%     tau = zeros(2,1);
% end

tau = zeros(2,1);

phi_tt = pendel.ode(phi, phi_t, pt_tt, l, l_t, g, c) + tau;

% add friction to pendulum
phi_tt = phi_tt;

end

== matlab function main/MotionLabSimulator/WEP in {n1} ==
  data: eta input; eta_t input; pt output; pt_t output; pt_tt output; eta_tt input; p input; p_t input; p_tt input
function [pt, pt_t, pt_tt] = fcn(eta, eta_t, eta_tt, p, p_t, p_tt)
    
    % Get body velocites
    [v, v_t] = math3d.eulerToBody(eta, eta_t, eta_tt, 'xyz');

    % Load Calibration data
    data = coder.load('motionlab/calib.mat');
    calib = data.calib;
    
    % Robot pose relative to EM8000
    Hbr = calib.EM8000_TO_COMAU.H;

    % Ship/stewart {b} orientation matrix relative to {n}
    Rnb = math3d.Rxyz(eta(4:6));

    % Body fixed velocity and acceleration skew matrices
    W = math3d.skew(v(4:6));
    W_t = math3d.skew(v_t(4:6));

    Rnb_t = Rnb*W;
    Rnb_tt = Rnb*W*W + Rnb*W_t;

    % Constant offsets {b} -> {r}
    r = Hbr(1:3,4);
    Rbr = Hbr(1:3,1:3);

    % Position of {t}/{n} given in {n}
    pt = eta(1:3) + Rnb*(r + Rbr*p);

    % Velocity of {t}/{n} given in {n}
    pt_t = v(1:3) + Rnb_t*(r + Rbr*p) + Rnb*(Rbr*p_t);

    % Acceleration of {t}/{n} given in {n}
    pt_tt = v_t(1:3) + Rnb_tt*(r + Rbr*p)...
        + 2*Rnb_t*(Rbr*p_t) + Rnb*(Rbr*p_tt);
end

== matlab function main/MotionLabSimulator/Winch Ode ==
  data: omega input; zeta input; l_ref input; l_tt output; l input; l_t input
function l_tt  = fcn(omega, zeta, l_ref, l, l_t)

l_tt = winch.ode(l_ref, l, l_t, omega, zeta);

end

== matlab function main/MotionLabSimulator/Robot Joint ODEs ==
  data: omega input; zeta input; q_ref input; q_tt output; q input; q_t input
function q_tt = fcn(omega, zeta,q_ref, q, q_t)


q_tt = joints.ode(q_ref, q, q_t, omega, zeta);


end

== matlab function main/MotionLabSimulator/Simulate Qualisys ==
  data: phi input; pt input; qtm output Bus: ST_FeedbackQualisys; l input; w input
function qtm = fcn(phi, pt, l, w)

data = coder.load('motionlab/calib.mat');
calib = data.calib;

% Get hook position in {n1}
ph = pendel.kinematics(pt, phi, l);

% Transform from {n1} to {g}
Hgq = calib.WORLD_TO_QTM.H;
Hgn = calib.WORLD_TO_EM8000.H;

Hqn = math3d.InvH(Hgq)*Hgn;

Ph = Hqn*[ph; 1];

% Return simulated qtm data
qtm.dist = 60/1000.0 + w(1)*1/1000;
qtm.pos = Ph(1:3) + w(2:4)*2/1000;

== matlab function main/MotionLabSimulator/FB_SimulateLeica ==
  data: em8000 input; at960 output Bus: ST_FeedbackLeica; em1500 input
function at960 = fcn(em8000, em1500)

data = coder.load('motionlab/calib.mat');
calib = data.calib;

% Stewart bodies
Hg1 = calib.WORLD_TO_EM8000.H*stewartToH(em8000);
Hg2 = calib.WORLD_TO_EM1500.H*stewartToH(em1500);

HgL = Hg1*calib.EM8000_TO_AT960.H;
HgP = Hg2*calib.EM1500_TO_TMAC.H;

% Leica measure
HLP = math3d.InvH(HgL)*HgP;

% Return simulated measurements
at960.pos = HLP(1:3,4);

at960.R11 = HLP(1,1);
at960.R12 = HLP(1,2);
at960.R13 = HLP(1,3);

at960.R21 = HLP(2,1);
at960.R22 = HLP(2,2);
at960.R23 = HLP(2,3);

at960.R31 = HLP(3,1);
at960.R32 = HLP(3,2);
at960.R33 = HLP(3,3);


end

function H = stewartToH(stewart)


H = eye(4);

H(1:3,4) = stewart.eta(1:3);
H(1:3,1:3) = math3d.Rxyz(stewart.eta(4:6));


end

== matlab function main/FB_WaveSimulator/zyx2xyz1 ==
  data: eta input; eta output
function eta = fcn(eta)

% Convert Angle sequence
eta(4:6) = math3d.zyx2xyz(eta(4:6));

end

== matlab function main/MotionLabSimulator/Feedback Simulator/MruEM8000/MruJacobian ==
  data: eta input; v output; eta_t input
function v = fcn(eta, eta_t)

% Velcoity Jacobian
J = eye(6);
J(4:6,4:6) = math3d.Tphi(eta(4:6), 'xyz');

% Body fixed velocities
v = J\eta_t;

end

== matlab function main/MotionLabSimulator/Feedback Simulator/EM1/Jacobian ==
  data: eta input; v output; eta_t input
function v  = fcn(eta, eta_t)

J = eye(6);

J(4:6,4:6) = math3d.Tphi(eta(4:6), 'xyz');

v = J\eta_t;

== matlab function main/MotionLabSimulator/Feedback Simulator/EM2/Jacobian ==
  data: eta input; v output; eta_t input
function v  = fcn(eta, eta_t)

J = eye(6);

J(4:6,4:6) = math3d.Tphi(eta(4:6), 'xyz');

v = J\eta_t;

== matlab function main/FB_ControlMapping ==
  data: useMru input; q0 input; q0_t input; p input; stControlComau output Bus: ST_ControlComau; p_t input; stFeedback input
function stControlComau = fcn(useMru, q0, q0_t, p, p_t, stFeedback)

% r1 = [q0; q0_t]

% EM8000 motion
if useMru
    eta = stFeedback.mru1.eta;
    v = stFeedback.mru1.v;
else
    eta = stFeedback.em8000.eta;
    eta_t = stFeedback.em8000.eta_t;
    
    [v, ~] = math3d.eulerToBody(eta, eta_t, zeros(6,1), 'xyz');
end

% Load Calibration data
data = coder.load('motionlab/calib.mat');
calib = data.calib;

Hbc = calib.EM8000_TO_COMAU.H;
Rbc = Hbc(1:3,1:3);

% Rotation matrices
Rnb = math3d.Rxyz(eta(4:6));
Rnb_t = Rnb*math3d.skew(v(4:6));

Rnc = Rnb*Rbc;
Rnc_t = Rnb_t*Rbc;

% Forward kinematics
[p0, p0_t, ~] = motionlab.comau.forward(q0, q0_t, zeros(3,1));

% Attitude corrected reference
AC = Rnc'*Rbc*p0;
AC_t = Rnc_t'*Rbc*p0 + Rnc'*Rbc*p0_t;

% LQR correction due to non zero swing angles
LQR = Rnc'*p;
LQR_t = Rnc_t'*p + Rnc'*p_t;

% Output u1 = [q; q_t]
[q, q_t, ~] = motionlab.comau.inverse(AC + LQR, AC_t + LQR_t, zeros(3,1));

% PLC data type
stControlComau.q = q;
stControlComau.q_t = q_t;
stControlComau.q_tt = zeros(3,1);


end

== matlab function main/FB_LqrAntiSwing/StackLqrStateVector ==
  data: active input; p_t input; p input; phi input; phi_t input; x output
function x  = fcn(active, p_t, p, phi, phi_t)

if active
    x = [
        p
        p_t
        phi
        phi_t
    ];
else
    x = [
        p
        p_t
        zeros(2,1)
        zeros(2,1)
    ];
end

end

== matlab function main/FB_PendelEKF/Discrete EKF ==
  data: pt output; pt_t output; pt_tt output; phi output; phi_t output; l output; l_t output; c output; e output; Ts input; diagQ input; diagR input; x output; z input; x input; P input; P output
function [pt, pt_t, pt_tt, phi, phi_t, l, l_t, c, e, x, P] = fcn(Ts, diagQ, diagR, z, x, P)

% Make Q and R
Q = diag(diagQ);
R = diag(diagR);

% Prediction
xPred = observer.f(x, Ts);
F = observer.fJacobian(x, Ts);
PPred = F*P*F' + Q;

% Measurement update
y = z - observer.h(xPred);

H = observer.hJacobian(xPred);
S = H*PPred*H' + R;

K = PPred*H'*inv(S);


x = xPred + K*y;
I = eye(length(x));
P = (I - K*H)*PPred;

% Convert from x -> variables
pt = x(1:3);
pt_t = x(4:6);
pt_tt = x(7:9);
phi = x(10:11);
phi_t = x(12:13);
l = x(14);
l_t = x(15);
c = x(16);
e = x(17:19);

end

== matlab function main/FB_QuatToRotMatrix ==
  data: w input; R11 output; x input; y input; z input; R12 output; R13 output; R21 output; R22 output; R23 output; R31 output; R32 output; R33 output
function [R11, R12, R13, R21, R22, R23, R31, R32, R33] = fcn(w, x, y, z)

quat = [w, x, y, z];

R = quat2rotm(quat);

R11 = R(1,1);
R12 = R(1,2);
R13 = R(1,3);

R21 = R(2,1);
R22 = R(2,2);
R23 = R(2,3);

R31 = R(3,1);
R32 = R(3,2);
R33 = R(3,3);

end

== matlab function main/FB_PendelEKF/VectorizeData ==
  data: feedback input Bus: ST_Feedback; z output; useMru input
function z  = fcn(feedback, useMru)


if useMru
    % Use 
    eta = feedback.mru1.eta;
    v = feedback.mru1.v;
else
    % Get body velocites
    eta = feedback.em8000.eta;
    eta_t = feedback.em8000.eta_t;

    [v, ~] = math3d.eulerToBody(eta, eta_t, zeros(6,1), 'xyz');
end

% Comau movement
q = feedback.comau.q;
q_t = feedback.comau.q_t;

[p, p_t, ~] = motionlab.comau.forward(q, q_t, zeros(3,1));

% Load Calibration data
data = coder.load('motionlab/calib.mat');
calib = data.calib;

% Robot pose relative to EM8000
Hbr = calib.EM8000_TO_COMAU.H;

% Ship/stewart {b} orientation matrix relative to {n}
Rnb = math3d.Rxyz(eta(4:6));

% Body fixed velocity and acceleration skew matrices
W = math3d.skew(v(4:6));

Rnb_t = Rnb*W;

% Constant offsets {b} -> {r}
r = Hbr(1:3,4);
Rbr = Hbr(1:3,1:3);

% Position of {t}/{n} given in {n}
pt = eta(1:3) + Rnb*(r + Rbr*p);

% Velocity of {t}/{n} given in {n}
pt_t = v(1:3) + Rnb_t*(r + Rbr*p) + Rnb*(Rbr*p_t);
    
% Hook measurement
ph = feedback.qtm.pos;
Hnq = math3d.InvH(calib.WORLD_TO_EM8000.H)*calib.WORLD_TO_QTM.H;
Ph = Hnq*[ph; 1];

z = [    
    pt
    pt_t
    feedback.winch.length
    feedback.winch.length_t
    Ph(1:3)
];



end

== matlab function main/FB_WinchController/Wire Length ==
  data: useMru input; h input; feedback input; d output; d_t output
function [d, d_t]  = fcn(useMru, h, feedback)

if useMru
    % Stack data from MRU
    eta1 = feedback.mru1.eta;
    v1 = feedback.mru1.v;

    eta2 = feedback.mru2.eta;
    v2 = feedback.mru2.v;
else
    % Use Stewart feedback
    eta1 = feedback.em8000.eta;
    eta1_t = feedback.em8000.eta_t; 
    [v1, ~] = math3d.eulerToBody(eta1, eta1_t, zeros(6,1), 'xyz');
   
    eta2 = feedback.em1500.eta;
    eta2_t = feedback.em1500.eta_t;
    [v2, ~] = math3d.eulerToBody(eta2, eta2_t, zeros(6,1), 'xyz');
end
    
% Comau angle feedback signals
q = feedback.comau.q;
q_t = feedback.comau.q_t;

% Comau forward kineamtics
[p, p_t, ~] = motionlab.comau.forward(q, q_t, zeros(3,1));

% Load calibration data
data = coder.load('motionlab/calib.mat');
calib = data.calib;

% Crane/robot location
Hbc = calib.EM8000_TO_COMAU.H;

% Heading offset
Hn1n2 = calib.EM8000_TO_EM1500.H;

Rn1b1 = math3d.Rxyz(eta1(4:6));
Rn1b1_t = Rn1b1*math3d.skew(v1(4:6));

Rn2b2 = math3d.Rxyz(eta2(4:6));
Rn2b2_t = Rn2b2*math3d.skew(v2(4:6));

% Tool in {n1}
rt = eta1(1:3) + Rn1b1*(Hbc(1:3,4) + Hbc(1:3,1:3)*p);
rt_t = v1(1:3) + Rn1b1_t*(Hbc(1:3,4) + Hbc(1:3,1:3)*p) + Rn1b1*Hbc(1:3,1:3)*p_t;

% Plane point pd in {n1}
r = [0; 0; h];
rd = Hn1n2(1:3,4) + Hn1n2(1:3,1:3)*(eta2(1:3) + Rn2b2*r);
rd_t = Hn1n2(1:3,1:3)*(v2(1:3) + Rn2b2_t*r);

% Vector w
w = rt - rd;
w_t = rt_t  - rd_t;

% Vector nd
Rn1b2 = Hn1n2(1:3,1:3)*Rn2b2;
Rn1b2_t = Hn1n2(1:3,1:3)*Rn2b2_t;

nd = -([0, 0, 1]*Rn1b2')';
nd_t = -([0, 0, 1]*Rn1b2_t')';

% Vector nz
nz = [0; 0; 1];

% a and a_t
a = dot(w, nd);
a_t = dot(w_t, nd) + dot(w, nd_t);

% b and b_t
b = dot(nz, nd);
b_t = dot(nz, nd_t);

% Calculate wire length
d = -a/b;
d_t = (a*b_t)/(b^2) - a_t/b;
end
